simulink model "positionControlBalancing"  (Simulink 9.0)
settings: Solver=FixedStepDiscrete  StartTime=0.0  StopTime="Config.SIMULATION_TIME "  FixedStep=Config.tStep  RelTol=1e-3  EnableMultiTasking=on
PostLoadFcn:
  | %% Try to open the static GUI
  | try
  | 
  |     staticGUI = simulinkStaticGUI;
  | 
  | end
InitFcn:
  | %% initialize the simulation
  | cd(fileparts(which(bdroot)));
  | initPositionControlBalancing;
  | 
  | %% Try to edit the GUI (the user may have already closed it)
  | try
  | 
  |     %% Update Start Button
  |     set(sl_synch_handles.startButton,'Backgroundcolor',[0.0,1.0,0.0]);
  |     set(sl_synch_handles.startButton,'Enable','on');
  | 
  | end
StartFcn:
  | %% Try to edit the GUI (the user may have already closed it)
  | try
  | 
  |     %% Update Start Button
  |     set(sl_synch_handles.startButton,'Backgroundcolor',[0.8,0.8,0.8]);
  |     set(sl_synch_handles.startButton,'Enable','off');
  | 
  |     %% Update Compile Button
  |     set(sl_synch_handles.compileButton,'Backgroundcolor',[0.8,0.8,0.8]);
  |     set(sl_synch_handles.compileButton,'Enable','off');
  | 
  |     %% Update Exit Button
  |     set(sl_synch_handles.exitButton,'Backgroundcolor',[0.8,0.8,0.8]);
  |     set(sl_synch_handles.exitButton,'Enable','off');
  | 
  | end
StopFcn:
  | %% stop the simulation
  | cd(fileparts(which(bdroot)));
  | stopPositionControlBalancing;
  | 
  | %% Try to edit the GUI (the user may have already closed it)
  | try
  | 
  |     %% Update Compile Button
  |     set(sl_synch_handles.compileButton,'Backgroundcolor',[1.0,0.6,0.0]);
  |     set(sl_synch_handles.compileButton,'Enable','on');
  | 
  |     %% Update Exit Button
  |     set(sl_synch_handles.exitButton,'Backgroundcolor',[0.0,1.0,1.0]);
  |     set(sl_synch_handles.exitButton,'Enable','on');
  | 
  | end
undefined symbols (not defined in the file or in its folder): Config, DiscIntNeverNeededParam, ROBOT_DOF, Sat
libraries: WBToolboxLibrary x28
CloseFcn:
  | %% Try to close the GUI (the user might have already closed it)
  | try
  | 
  |     close(simulinkStaticGUI)
  | 
  | end
settings Model: SuppressorTable=22 serialization::archive 11 0 6 0 0 0 1 0  Creator=daniele  LastModifiedBy=gnava
settings DataIOCC: LimitDataPoints=on
settings OptimizationCC: ExpressionDepthLimit=2147483647
settings DebuggingCC: SolverPrmCheckMsg=warning  FcnCallInpInsideContextMsg=warning  AllowSymbolicDim=off  StateNameClashWarn=warning
settings SFSimCC: SimParseCustomCode=off
settings RTWCC: GenCodeOnly=on  TargetLang=C++
settings GRTTargetCC: TargetLangStandard=C++03 (ISO)  GeneratePreprocessorConditionals=Disable all  MatFileLogging=off  MultiInstanceERTCode=on  CodeInterfacePackaging=C++ class  SupportNonFinite=off
settings CPPComponent: GenerateDestructor=on  GenerateExternalIOAccessMethods=None  ParameterMemberVisibility=private  InternalMemberVisibility=private  GenerateParameterAccessMethods=None  GenerateInternalMemberAccessMethods=None  UseOperatorNewForModelRefRegistration=off

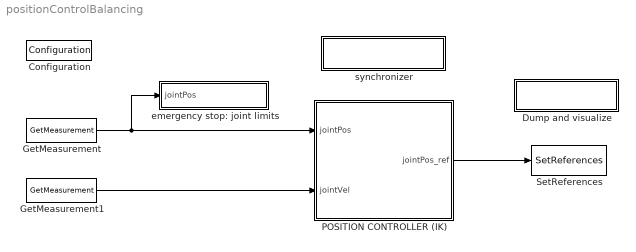
== system positionControlBalancing ==
  Configuration : WBToolboxLibrary/Utilities/Configuration  ConfigSource=Workspace  ConfigObject='WBTConfigRobot'  RobotName='icubSim'  UrdfFile='model.urdf'  ControlledJoints={'l_elbow','l_shoulder_pitch','torso_roll'}  ControlBoardsNames={'left_arm','right_arm','torso'}  LocalName='WBT'  GravityVector=[0,0,-9.81]
      settings: SourceProductName=WholeBodyToolbox
  Dump and visualize : Subsystem
      mask Display: disp('VISUALIZER')
  GetMeasurement : WBToolboxLibrary/States/GetMeasurement  measuredType=Joints Position
      settings: SourceProductName=WholeBodyToolbox
  GetMeasurement1 : WBToolboxLibrary/States/GetMeasurement  measuredType=Joints Velocity
      settings: SourceProductName=WholeBodyToolbox
  POSITION CONTROLLER (IK) : Subsystem
  SetReferences : WBToolboxLibrary/Actuators/SetReferences  controlType=Position Direct  refSpeed=10*(pi/180)  refAcceleration=1000000*(pi/180)
      settings: SourceProductName=WholeBodyToolbox
  emergency stop: joint limits : Subsystem
      mask Display: disp('EMERGENCY STOP')
  synchronizer : Subsystem
      mask Display: disp('SYNCHRONIZER')
  wires:
  POSITION CONTROLLER (IK)/1(jointPos_ref) -> SetReferences/1
  GetMeasurement/1 -> POSITION CONTROLLER (IK)/1(jointPos), emergency stop: joint limits/1(jointPos)
  GetMeasurement1/1 -> POSITION CONTROLLER (IK)/2(jointVel)

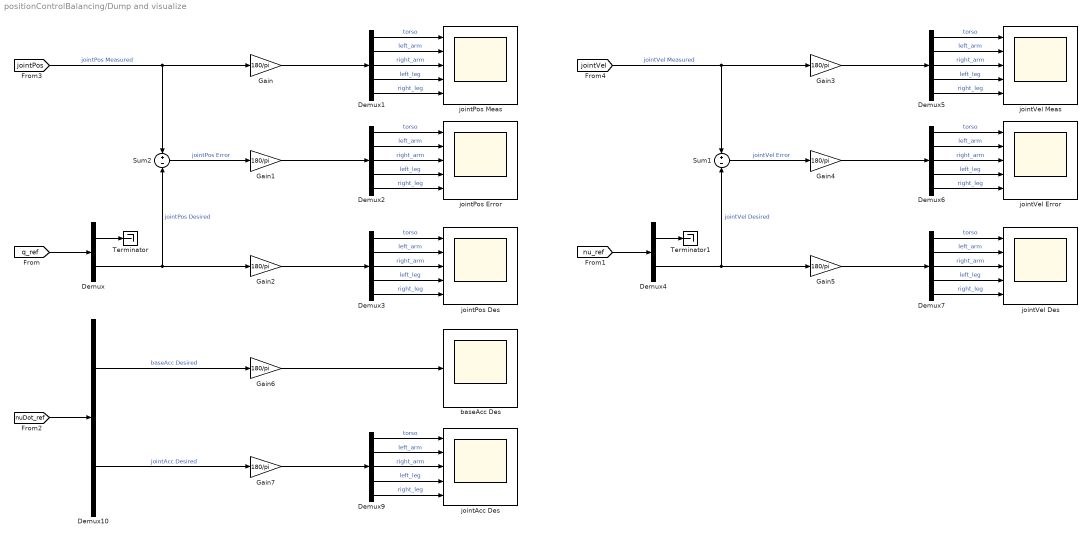
== system positionControlBalancing/Dump and visualize ==
  Demux : Demux  Outputs=[16;ROBOT_DOF]
  Demux{1..3,5..7,9} (7 alike) : Demux  Outputs=Config.numOfJointsForEachControlboard
  Demux10 : Demux  Outputs=[6;ROBOT_DOF]
  Demux4 : Demux  Outputs=[6;ROBOT_DOF]
  Gain{,1..7} (8 alike) : Gain  Gain=180/pi
  Sum1 : Sum  Inputs=+|-
  Sum2 : Sum  Inputs=+|-
  Terminator : Terminator
  Terminator1 : Terminator
  baseAcc Des : Scope
  jointAcc Des : Scope  NumInputPorts=5
  jointPos Des : Scope  NumInputPorts=5
  jointPos Error : Scope  NumInputPorts=5
  jointPos Meas : Scope  NumInputPorts=5
  jointVel Des : Scope  NumInputPorts=5
  jointVel Error : Scope  NumInputPorts=5
  jointVel Meas : Scope  NumInputPorts=5
  wires:
  Demux3/4 -> jointPos Des/4  "left_leg"
  Gain2/1 -> Demux3/1
  Demux2/5 -> jointPos Error/5  "right_leg"
  Demux2/4 -> jointPos Error/4  "left_leg"
  Demux3/1 -> jointPos Des/1  "torso"
  Demux3/5 -> jointPos Des/5  "right_leg"
  Demux1/3 -> jointPos Meas/3  "right_arm"
  Demux/2 -> Gain2/1, Sum2/2  "jointPos Desired"
  Gain1/1 -> Demux2/1
  Demux1/5 -> jointPos Meas/5  "right_leg"
  Demux1/1 -> jointPos Meas/1  "torso"
  Demux2/1 -> jointPos Error/1  "torso"
  Demux2/2 -> jointPos Error/2  "left_arm"
  Demux2/3 -> jointPos Error/3  "right_arm"
  Demux3/3 -> jointPos Des/3  "right_arm"
  Demux3/2 -> jointPos Des/2  "left_arm"
  Sum2/1 -> Gain1/1  "jointPos Error"
  Demux1/2 -> jointPos Meas/2  "left_arm"
  Gain/1 -> Demux1/1
  [jointPos] -> Sum2/1, Gain/1  "jointPos Measured"
  Demux1/4 -> jointPos Meas/4  "left_leg"
  [q_ref] -> Demux/1
  Demux/1 -> Terminator/1
  Demux4/1 -> Terminator1/1
  Demux6/2 -> jointVel Error/2  "left_arm"
  Demux6/3 -> jointVel Error/3  "right_arm"
  [jointVel] -> Sum1/1, Gain3/1  "jointVel Measured"
  Demux7/5 -> jointVel Des/5  "right_leg"
  Demux5/1 -> jointVel Meas/1  "torso"
  Demux7/4 -> jointVel Des/4  "left_leg"
  Demux6/4 -> jointVel Error/4  "left_leg"
  Sum1/1 -> Gain4/1  "jointVel Error"
  Demux7/3 -> jointVel Des/3  "right_arm"
  Demux4/2 -> Gain5/1, Sum1/2  "jointVel Desired"
  Demux6/5 -> jointVel Error/5  "right_leg"
  Demux5/2 -> jointVel Meas/2  "left_arm"
  Gain3/1 -> Demux5/1
  Demux5/3 -> jointVel Meas/3  "right_arm"
  [nu_ref] -> Demux4/1
  Demux7/1 -> jointVel Des/1  "torso"
  Demux6/1 -> jointVel Error/1  "torso"
  Gain5/1 -> Demux7/1
  Demux5/5 -> jointVel Meas/5  "right_leg"
  Gain4/1 -> Demux6/1
  Demux7/2 -> jointVel Des/2  "left_arm"
  Demux5/4 -> jointVel Meas/4  "left_leg"
  Demux10/1 -> Gain6/1  "baseAcc Desired"
  Gain7/1 -> Demux9/1
  Demux9/4 -> jointAcc Des/4  "left_leg"
  Demux9/3 -> jointAcc Des/3  "right_arm"
  Demux9/2 -> jointAcc Des/2  "left_arm"
  Demux9/5 -> jointAcc Des/5  "right_leg"
  Demux9/1 -> jointAcc Des/1  "torso"
  Demux10/2 -> Gain7/1  "jointAcc Desired"
  [nuDot_ref] -> Demux10/1
  Gain6/1 -> baseAcc Des/1

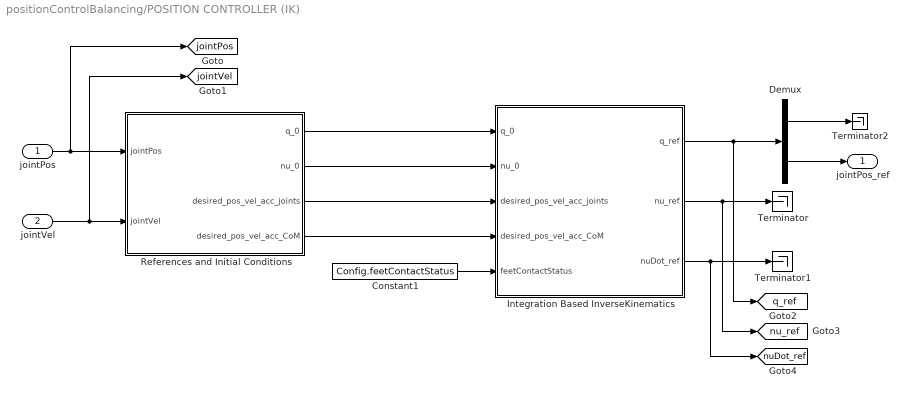
== system positionControlBalancing/POSITION CONTROLLER (IK) ==
  jointPos : Inport
  jointVel : Inport  Port=2
  Constant1 : Constant  Value=Config.feetContactStatus
  Demux : Demux  Outputs=[16;ROBOT_DOF]
  Integration Based InverseKinematics : Subsystem
  References and Initial Conditions : Subsystem
  Terminator : Terminator
  Terminator1 : Terminator
  Terminator2 : Terminator
  jointPos_ref : Outport
  tag scope: jointPos=global, jointVel=global, nuDot_ref=global, nu_ref=global, q_ref=global
  wires:
  jointPos/1 -> [jointPos], References and Initial Conditions/1(jointPos)
  jointVel/1 -> [jointVel], References and Initial Conditions/2(jointVel)
  References and Initial Conditions/1(q_0) -> Integration Based InverseKinematics/1(q_0)
  References and Initial Conditions/2(nu_0) -> Integration Based InverseKinematics/2(nu_0)
  References and Initial Conditions/3(desired_pos_vel_acc_joints) -> Integration Based InverseKinematics/3(desired_pos_vel_acc_joints)
  References and Initial Conditions/4(desired_pos_vel_acc_CoM) -> Integration Based InverseKinematics/4(desired_pos_vel_acc_CoM)
  Constant1/1 -> Integration Based InverseKinematics/5(feetContactStatus)
  Integration Based InverseKinematics/2(nu_ref) -> [nu_ref], Terminator/1
  Integration Based InverseKinematics/3(nuDot_ref) -> [nuDot_ref], Terminator1/1
  Integration Based InverseKinematics/1(q_ref) -> [q_ref], Demux/1
  Demux/1 -> Terminator2/1
  Demux/2 -> jointPos_ref/1

== system positionControlBalancing/emergency stop: joint limits ==
  jointPos : Inport
  ON_GAZEBO 1 : Constant  Value=Config.EMERGENCY_STOP_WITH_JOINTS_LIMITS
  ON_GAZEBO 2 : Constant  Value=Config.EMERGENCY_STOP_WITH_ENCODER_SPIKES
  STOP IF JOINTS HIT THE LIMITS : Subsystem
  STOP IF THERE ARE SPIKES IN THE ENCODERS : Subsystem
  wires:
  ON_GAZEBO 1/1 -> STOP IF JOINTS HIT THE LIMITS/Enable
  jointPos/1 -> STOP IF THERE ARE SPIKES IN THE ENCODERS/1(jointPos), STOP IF JOINTS HIT THE LIMITS/1(jointPos)
  ON_GAZEBO 2/1 -> STOP IF THERE ARE SPIKES IN THE ENCODERS/Enable

== system positionControlBalancing/synchronizer ==
  GAZEBO_SYNCHRONIZER : Subsystem
  Logical Operator : Logic  Operator=NOT  AllPortsSameDT=off  OutDataTypeStr=boolean
  "ON_GAZEBO " : Constant  Value=Config.ON_GAZEBO
  REAL_TIME_SYNC : Subsystem
  To Workspace : ToWorkspace  VariableName=yarp_time  SaveFormat=Structure With Time  SampleTime=-1
  Yarp Clock : WBToolboxLibrary/Utilities/Yarp Clock
      settings: SourceProductName=WholeBodyToolbox
  wires:
  Logical Operator/1 -> REAL_TIME_SYNC/Enable
  "ON_GAZEBO "/1 -> GAZEBO_SYNCHRONIZER/Enable, Logical Operator/1
  Yarp Clock/1 -> To Workspace/1

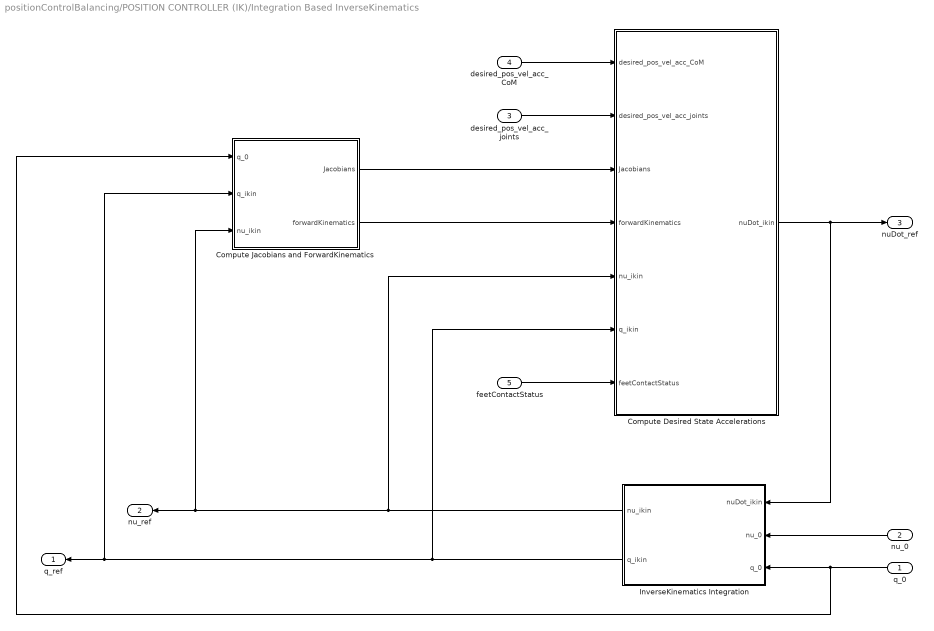
== system positionControlBalancing/POSITION CONTROLLER (IK)/Integration Based InverseKinematics ==
  q_0 : Inport
  nu_0 : Inport  Port=2
  desired_pos_vel_acc_joints : Inport  Port=3
  desired_pos_vel_acc_CoM : Inport  Port=4
  feetContactStatus : Inport  Port=5
  Compute Desired State Accelerations : Subsystem
  Compute Jacobians and ForwardKinematics : Subsystem
  InverseKinematics Integration : Subsystem
  q_ref : Outport
  nu_ref : Outport  Port=2
  nuDot_ref : Outport  Port=3
  wires:
  desired_pos_vel_acc_CoM/1 -> Compute Desired State Accelerations/1(desired_pos_vel_acc_CoM)
  desired_pos_vel_acc_joints/1 -> Compute Desired State Accelerations/2(desired_pos_vel_acc_joints)
  q_0/1 -> Compute Jacobians and ForwardKinematics/1(q_0), InverseKinematics Integration/3(q_0)
  InverseKinematics Integration/2(q_ikin) -> q_ref/1, Compute Jacobians and ForwardKinematics/2(q_ikin), Compute Desired State Accelerations/6(q_ikin)
  Compute Jacobians and ForwardKinematics/1(Jacobians) -> Compute Desired State Accelerations/3(Jacobians)
  Compute Jacobians and ForwardKinematics/2(forwardKinematics) -> Compute Desired State Accelerations/4(forwardKinematics)
  Compute Desired State Accelerations/1(nuDot_ikin) -> InverseKinematics Integration/1(nuDot_ikin), nuDot_ref/1
  feetContactStatus/1 -> Compute Desired State Accelerations/7(feetContactStatus)
  nu_0/1 -> InverseKinematics Integration/2(nu_0)
  InverseKinematics Integration/1(nu_ikin) -> nu_ref/1, Compute Jacobians and ForwardKinematics/3(nu_ikin), Compute Desired State Accelerations/5(nu_ikin)

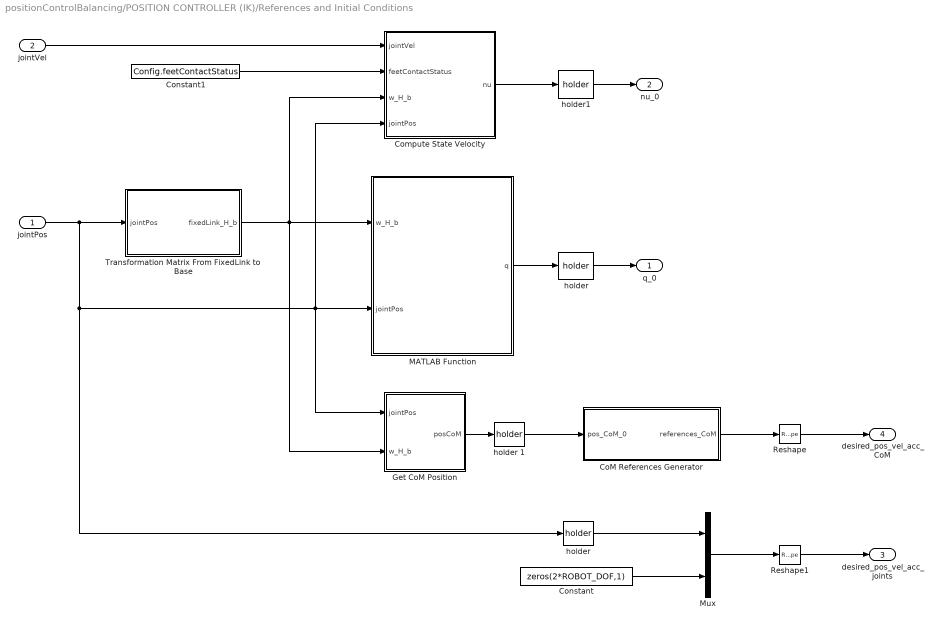
== system positionControlBalancing/POSITION CONTROLLER (IK)/References and Initial Conditions ==
  jointPos : Inport
  jointVel : Inport  Port=2
  CoM References Generator : Subsystem
  Compute State Velocity : Subsystem
  Constant : Constant  Value=zeros(2*ROBOT_DOF,1)
  Constant1 : Constant  Value=Config.feetContactStatus
  Get CoM Position : Subsystem
  MATLAB Function : MATLAB Function  TreatAsAtomicUnit=on
  Mux : Mux  Inputs=2
  Reshape : Reshape  OutputDimensionality=Customize  OutputDimensions=[3,3]
  Reshape1 : Reshape  OutputDimensionality=Customize  OutputDimensions=[ROBOT_DOF,3]
  Transformation Matrix From FixedLink to Base : Subsystem
  holder : WBToolboxLibrary/Utilities/holder 
      settings: SourceProductName=WholeBodyToolbox
  "holder " : WBToolboxLibrary/Utilities/holder 
      settings: SourceProductName=WholeBodyToolbox
  holder 1 : WBToolboxLibrary/Utilities/holder 
      settings: SourceProductName=WholeBodyToolbox
  holder1 : WBToolboxLibrary/Utilities/holder 
      settings: SourceProductName=WholeBodyToolbox
  q_0 : Outport
  nu_0 : Outport  Port=2
  desired_pos_vel_acc_joints : Outport  Port=3
  desired_pos_vel_acc_CoM : Outport  Port=4
  wires:
  CoM References Generator/1(references_CoM) -> Reshape/1
  Compute State Velocity/1(nu) -> holder1/1
  Get CoM Position/1(posCoM) -> holder 1/1
  Constant1/1 -> Compute State Velocity/2("feetContactStatus ")
  Reshape/1 -> desired_pos_vel_acc_CoM/1
  holder 1/1 -> CoM References Generator/1(pos_CoM_0)
  Transformation Matrix From FixedLink to Base/1(fixedLink_H_b) -> Get CoM Position/2(w_H_b), Compute State Velocity/3(w_H_b), MATLAB Function/1(w_H_b)
  MATLAB Function/1(q) -> holder/1
  jointPos/1 -> Transformation Matrix From FixedLink to Base/1(jointPos), "holder "/1, Get CoM Position/1(jointPos), Compute State Velocity/4(jointPos), MATLAB Function/2(jointPos)
  holder/1 -> q_0/1
  jointVel/1 -> Compute State Velocity/1(jointVel)
  holder1/1 -> nu_0/1
  Constant/1 -> Mux/2
  "holder "/1 -> Mux/1
  Mux/1 -> Reshape1/1
  Reshape1/1 -> desired_pos_vel_acc_joints/1

== system positionControlBalancing/emergency stop: joint limits/STOP IF JOINTS HIT THE LIMITS ==
  jointPos : Inport
  Enable : EnablePort
  Assertion : Assertion
  GetLimits : WBToolboxLibrary/States/GetLimits  limitsSource=ControlBoard  limitsType=Position
      settings: SourceProductName=WholeBodyToolbox
  MATLAB Function : MATLAB Function  TreatAsAtomicUnit=on
  index1 : Constant  Value=0.01  VectorParams1D=off
  wires:
  jointPos/1 -> MATLAB Function/3(u)
  MATLAB Function/1(inRange) -> Assertion/1
  GetLimits/1 -> MATLAB Function/1(umin)
  GetLimits/2 -> MATLAB Function/2(umax)
  index1/1 -> MATLAB Function/4(tol)

== system positionControlBalancing/emergency stop: joint limits/STOP IF THERE ARE SPIKES IN THE ENCODERS ==
  jointPos : Inport
  Enable : EnablePort
  Assertion : Assertion
  MATLAB Function : MATLAB Function  TreatAsAtomicUnit=on
  index1 : Constant  Value=Sat.maxJointsPositionDelta  VectorParams1D=off
  wires:
  jointPos/1 -> MATLAB Function/1(u)
  MATLAB Function/1(noSpikes) -> Assertion/1
  index1/1 -> MATLAB Function/2(delta_u_max)

== system positionControlBalancing/synchronizer/GAZEBO_SYNCHRONIZER ==
  Enable : EnablePort
  Simulator Synchronizer : WBToolboxLibrary/Utilities/Simulator Synchronizer  period=Config.tStep  serverPortName='/clock/rpc'  clientPortName='/WBT_synchronizer/rpc:o'
      settings: SourceProductName=WholeBodyToolbox

== system positionControlBalancing/synchronizer/REAL_TIME_SYNC ==
  Enable : EnablePort
  Real Time Synchronizer : WBToolboxLibrary/Utilities/Real Time Synchronizer  period=Config.tStep
      settings: SourceProductName=WholeBodyToolbox

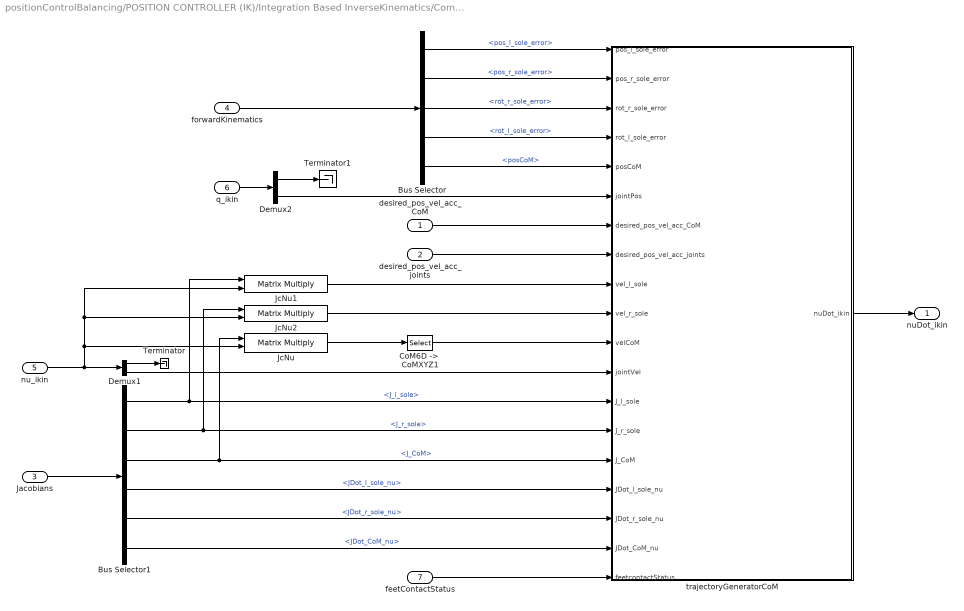
== system positionControlBalancing/POSITION CONTROLLER (IK)/Integration Based InverseKinematics/Compute Desired State Accelerations ==
  desired_pos_vel_acc_CoM : Inport
  desired_pos_vel_acc_joints : Inport  Port=2
  Jacobians : Inport  Port=3
  forwardKinematics : Inport  Port=4
  nu_ikin : Inport  Port=5
  q_ikin : Inport  Port=6
  feetContactStatus : Inport  Port=7
  Bus Selector : BusSelector  OutputSignals=pos_l_sole_error,pos_r_sole_error,rot_r_sole_error,rot_l_sole_error,posCoM
  Bus Selector1 : BusSelector  OutputSignals=J_l_sole,J_r_sole,J_CoM,JDot_l_sole_nu,JDot_r_sole_nu,JDot_CoM_nu
  "CoM6D ->  CoMXYZ1" : Selector  InputPortWidth=6  IndexOptions=Index vector (dialog)  Indices=[1 2 3]  OutputSizes=1
  Demux1 : Demux  Outputs=[6,ROBOT_DOF]
  Demux2 : Demux  Outputs=[16,ROBOT_DOF]
  JcNu : Product  Multiplication=Matrix(*)
  JcNu1 : Product  Multiplication=Matrix(*)
  JcNu2 : Product  Multiplication=Matrix(*)
  Terminator : Terminator
  Terminator1 : Terminator
  trajectoryGeneratorCoM : MATLAB Function  TreatAsAtomicUnit=on
  nuDot_ikin : Outport
  wires:
  Demux1/1 -> Terminator/1
  JcNu/1 -> "CoM6D ->  CoMXYZ1"/1
  q_ikin/1 -> Demux2/1
  Demux2/1 -> Terminator1/1
  trajectoryGeneratorCoM/1(nuDot_ikin) -> nuDot_ikin/1
  desired_pos_vel_acc_CoM/1 -> trajectoryGeneratorCoM/7(desired_pos_vel_acc_CoM)
  desired_pos_vel_acc_joints/1 -> trajectoryGeneratorCoM/8(desired_pos_vel_acc_joints)
  feetContactStatus/1 -> trajectoryGeneratorCoM/19(feetcontactStatus)
  nu_ikin/1 -> JcNu1/2, JcNu2/2, JcNu/2, Demux1/1
  forwardKinematics/1 -> Bus Selector/1
  Bus Selector/1 -> trajectoryGeneratorCoM/1(pos_l_sole_error)  "<pos_l_sole_error>"
  Bus Selector/2 -> trajectoryGeneratorCoM/2(pos_r_sole_error)  "<pos_r_sole_error>"
  Bus Selector/3 -> trajectoryGeneratorCoM/3(rot_r_sole_error)  "<rot_r_sole_error>"
  Bus Selector/4 -> trajectoryGeneratorCoM/4(rot_l_sole_error)  "<rot_l_sole_error>"
  Bus Selector/5 -> trajectoryGeneratorCoM/5(posCoM)  "<posCoM>"
  Demux2/2 -> trajectoryGeneratorCoM/6(jointPos)
  Jacobians/1 -> Bus Selector1/1
  Bus Selector1/1 -> JcNu1/1, trajectoryGeneratorCoM/13(J_l_sole)  "<J_l_sole>"
  Bus Selector1/2 -> JcNu2/1, trajectoryGeneratorCoM/14(J_r_sole)  "<J_r_sole>"
  Bus Selector1/3 -> JcNu/1, trajectoryGeneratorCoM/15(J_CoM)  "<J_CoM>"
  Bus Selector1/4 -> trajectoryGeneratorCoM/16(JDot_l_sole_nu)  "<JDot_l_sole_nu>"
  Bus Selector1/5 -> trajectoryGeneratorCoM/17(JDot_r_sole_nu)  "<JDot_r_sole_nu>"
  Bus Selector1/6 -> trajectoryGeneratorCoM/18(JDot_CoM_nu)  "<JDot_CoM_nu>"
  JcNu1/1 -> trajectoryGeneratorCoM/9(vel_l_sole)
  JcNu2/1 -> trajectoryGeneratorCoM/10(vel_r_sole)
  "CoM6D ->  CoMXYZ1"/1 -> trajectoryGeneratorCoM/11(velCoM)
  Demux1/2 -> trajectoryGeneratorCoM/12(jointVel)

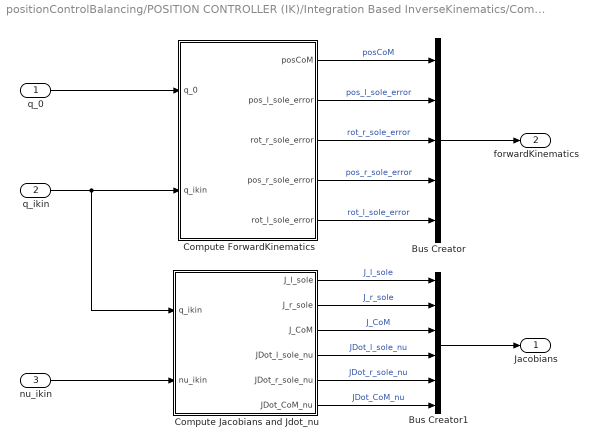
== system positionControlBalancing/POSITION CONTROLLER (IK)/Integration Based InverseKinematics/Compute Jacobians and ForwardKinematics ==
  q_0 : Inport
  q_ikin : Inport  Port=2
  nu_ikin : Inport  Port=3
  Bus Creator : BusCreator  Inputs=5
  Bus Creator1 : BusCreator  Inputs=6
  Compute ForwardKinematics : Subsystem
  Compute Jacobians and Jdot_nu : Subsystem
  Jacobians : Outport
  forwardKinematics : Outport  Port=2
  wires:
  q_0/1 -> Compute ForwardKinematics/1(q_0)
  q_ikin/1 -> Compute Jacobians and Jdot_nu/1(q_ikin), Compute ForwardKinematics/2(q_ikin)
  Compute ForwardKinematics/1(posCoM) -> Bus Creator/1  "posCoM"
  Compute ForwardKinematics/2(pos_l_sole_error) -> Bus Creator/2  "pos_l_sole_error"
  Compute ForwardKinematics/3(rot_r_sole_error) -> Bus Creator/3  "rot_r_sole_error"
  Compute ForwardKinematics/4(pos_r_sole_error) -> Bus Creator/4  "pos_r_sole_error"
  Compute ForwardKinematics/5(rot_l_sole_error) -> Bus Creator/5  "rot_l_sole_error"
  Bus Creator/1 -> forwardKinematics/1
  nu_ikin/1 -> Compute Jacobians and Jdot_nu/2(nu_ikin)
  Compute Jacobians and Jdot_nu/1(J_l_sole) -> Bus Creator1/1  "J_l_sole"
  Compute Jacobians and Jdot_nu/2(J_r_sole) -> Bus Creator1/2  "J_r_sole"
  Compute Jacobians and Jdot_nu/3(J_CoM) -> Bus Creator1/3  "J_CoM"
  Compute Jacobians and Jdot_nu/4(JDot_l_sole_nu) -> Bus Creator1/4  "JDot_l_sole_nu"
  Compute Jacobians and Jdot_nu/5(JDot_r_sole_nu) -> Bus Creator1/5  "JDot_r_sole_nu"
  Compute Jacobians and Jdot_nu/6(JDot_CoM_nu) -> Bus Creator1/6  "JDot_CoM_nu"
  Bus Creator1/1 -> Jacobians/1

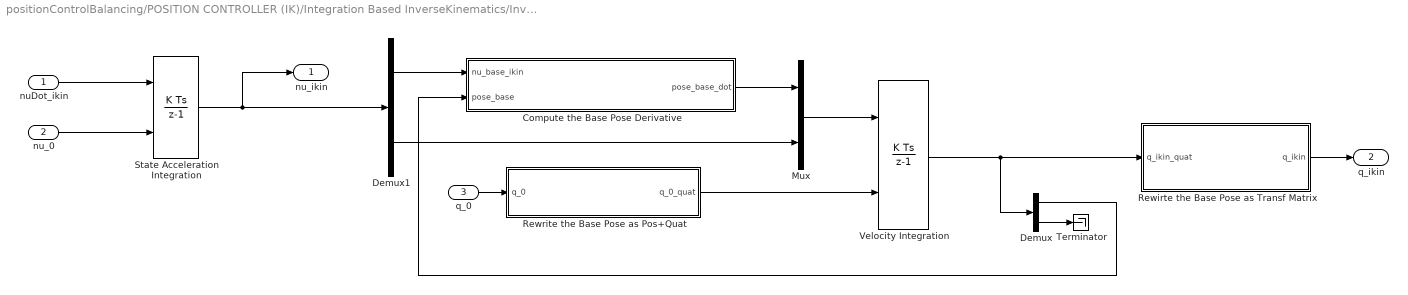
== system positionControlBalancing/POSITION CONTROLLER (IK)/Integration Based InverseKinematics/InverseKinematics Integration ==
  nuDot_ikin : Inport
  nu_0 : Inport  Port=2
  q_0 : Inport  Port=3
  Compute the Base Pose Derivative : MATLAB Function  TreatAsAtomicUnit=on
  Demux : Demux  Outputs=[7;ROBOT_DOF]
  Demux1 : Demux  Outputs=[6;ROBOT_DOF]
  Mux : Mux  Inputs=2
  Rewirte the Base Pose as Transf Matrix : MATLAB Function  TreatAsAtomicUnit=on
  Rewrite the Base Pose as Pos+Quat : MATLAB Function  TreatAsAtomicUnit=on
  State Acceleration Integration : DiscreteIntegrator  InitialConditionSource=external  SampleTime=Config.tStep  ICPrevOutput=DiscIntNeverNeededParam  ICPrevScaledInput=DiscIntNeverNeededParam
  Terminator : Terminator
  Velocity Integration : DiscreteIntegrator  InitialConditionSource=external  SampleTime=Config.tStep  ICPrevOutput=DiscIntNeverNeededParam  ICPrevScaledInput=DiscIntNeverNeededParam
  nu_ikin : Outport
  q_ikin : Outport  Port=2
  wires:
  nu_0/1 -> State Acceleration Integration/2
  q_0/1 -> Rewrite the Base Pose as Pos+Quat/1(q_0)
  nuDot_ikin/1 -> State Acceleration Integration/1
  Demux/2 -> Terminator/1
  Velocity Integration/1 -> Demux/1, Rewirte the Base Pose as Transf Matrix/1(q_ikin_quat)
  State Acceleration Integration/1 -> Demux1/1, nu_ikin/1
  Demux1/1 -> Compute the Base Pose Derivative/1(nu_base_ikin)
  Compute the Base Pose Derivative/1(pose_base_dot) -> Mux/1
  Demux1/2 -> Mux/2
  Mux/1 -> Velocity Integration/1
  Rewirte the Base Pose as Transf Matrix/1(q_ikin) -> q_ikin/1
  Rewrite the Base Pose as Pos+Quat/1(q_0_quat) -> Velocity Integration/2
  Demux/1 -> Compute the Base Pose Derivative/2(pose_base)

== system positionControlBalancing/POSITION CONTROLLER (IK)/References and Initial Conditions/CoM References Generator ==
  pos_CoM_0 : Inport
  Clock1 : Clock
  Constant : Constant  Value=Config.COM_SINE_MOVEMENTS
  Constant2 : Constant  Value=zeros(6,1)
  Mux : Mux  Inputs=2
  Reference Generator CoM : MATLAB Function  TreatAsAtomicUnit=on
  Switch1 : Switch  Criteria=u2 > Threshold
  references_CoM : Outport
  wires:
  Clock1/1 -> Reference Generator CoM/2(t)
  Constant2/1 -> Mux/2
  pos_CoM_0/1 -> Reference Generator CoM/1(posCoM_0), Mux/1
  Constant/1 -> Switch1/2
  Mux/1 -> Switch1/3
  Reference Generator CoM/1(references_CoM) -> Switch1/1
  Switch1/1 -> references_CoM/1

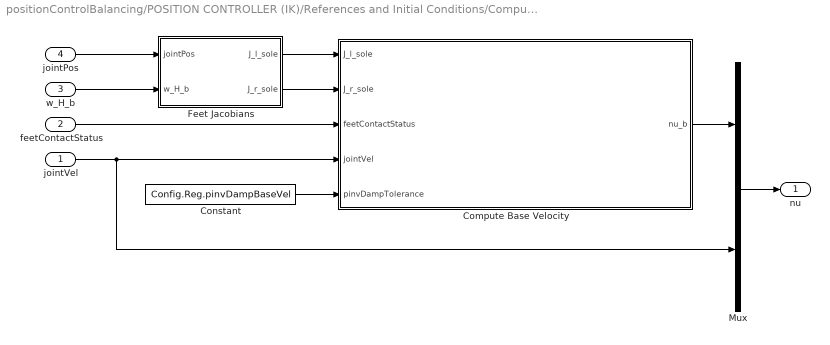
== system positionControlBalancing/POSITION CONTROLLER (IK)/References and Initial Conditions/Compute State Velocity ==
  jointVel : Inport
  "feetContactStatus " : Inport  Port=2
  w_H_b : Inport  Port=3
  jointPos : Inport  Port=4
  Compute Base Velocity : MATLAB Function  TreatAsAtomicUnit=on
  Constant : Constant  Value=Config.Reg.pinvDampBaseVel
  Feet Jacobians : Subsystem
  Mux : Mux  Inputs=2
  nu : Outport
  wires:
  Mux/1 -> nu/1
  "feetContactStatus "/1 -> Compute Base Velocity/3(feetContactStatus)
  Compute Base Velocity/1(nu_b) -> Mux/1
  jointPos/1 -> Feet Jacobians/1(jointPos)
  w_H_b/1 -> Feet Jacobians/2(w_H_b)
  Feet Jacobians/1(J_l_sole) -> Compute Base Velocity/1(J_l_sole)
  Feet Jacobians/2(J_r_sole) -> Compute Base Velocity/2(J_r_sole)
  jointVel/1 -> Compute Base Velocity/4(jointVel), Mux/2
  Constant/1 -> Compute Base Velocity/5(pinvDampTolerance)

== system positionControlBalancing/POSITION CONTROLLER (IK)/References and Initial Conditions/Get CoM Position ==
  jointPos : Inport
  w_H_b : Inport  Port=2
  CoM Position : WBToolboxLibrary/Model/Kinematics/ForwardKinematics  frameName=Frames.COM
      settings: SourceProductName=WholeBodyToolbox
  "CoM6D ->  CoMXYZ2" : Selector  NumberOfDimensions=2  InputPortWidth=7  IndexOptions=Index vector (dialog),Index vector (dialog)  Indices=[1 2 3],[4]  OutputSizes=1,1
  posCoM : Outport
  wires:
  jointPos/1 -> CoM Position/2
  "CoM6D ->  CoMXYZ2"/1 -> posCoM/1
  CoM Position/1 -> "CoM6D ->  CoMXYZ2"/1
  w_H_b/1 -> CoM Position/1

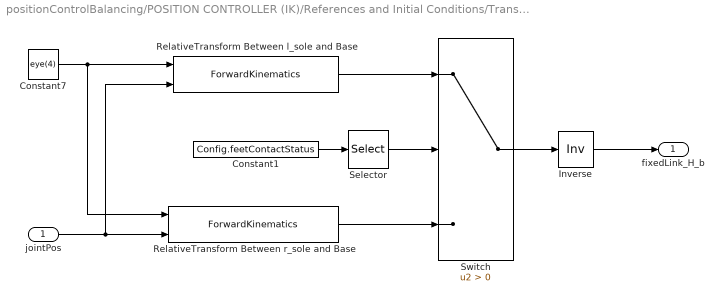
== system positionControlBalancing/POSITION CONTROLLER (IK)/References and Initial Conditions/Transformation Matrix From FixedLink to Base ==
  jointPos : Inport
  Constant1 : Constant  Value=Config.feetContactStatus
  Constant7 : Constant  Value=eye(4)
  "Inverse  " : Product  Inputs=/  Multiplication=Matrix(*)
  RelativeTransform Between l_sole and Base : WBToolboxLibrary/Model/Kinematics/ForwardKinematics  frameName=Frames.LEFT_FOOT
      settings: SourceProductName=WholeBodyToolbox
  RelativeTransform Between r_sole and Base : WBToolboxLibrary/Model/Kinematics/ForwardKinematics  frameName=Frames.RIGHT_FOOT
      settings: SourceProductName=WholeBodyToolbox
  Selector : Selector  InputPortWidth=2  IndexOptions=Index vector (dialog)  Indices=1  OutputSizes=1
  Switch : Switch  Criteria=u2 > Threshold
  fixedLink_H_b : Outport
  wires:
  jointPos/1 -> RelativeTransform Between l_sole and Base/2, RelativeTransform Between r_sole and Base/2
  Constant7/1 -> RelativeTransform Between r_sole and Base/1, RelativeTransform Between l_sole and Base/1
  RelativeTransform Between l_sole and Base/1 -> Switch/1
  RelativeTransform Between r_sole and Base/1 -> Switch/3
  Constant1/1 -> Selector/1
  Switch/1 -> "Inverse  "/1
  "Inverse  "/1 -> fixedLink_H_b/1
  Selector/1 -> Switch/2

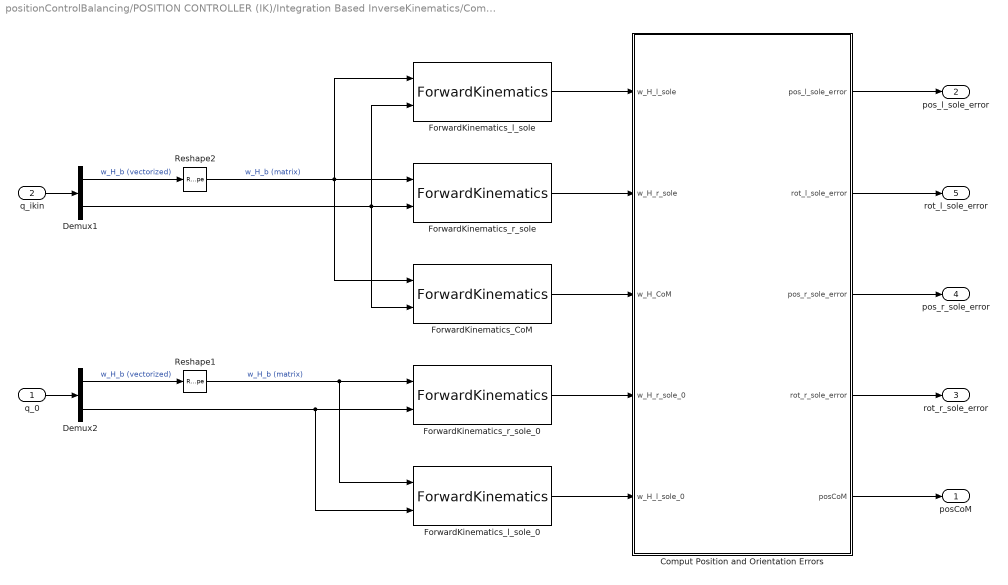
== system positionControlBalancing/POSITION CONTROLLER (IK)/Integration Based InverseKinematics/Compute Jacobians and ForwardKinematics/Compute ForwardKinematics ==
  q_0 : Inport
  q_ikin : Inport  Port=2
  Comput Position and Orientation Errors : MATLAB Function  TreatAsAtomicUnit=on
  Demux1 : Demux  Outputs=[16;ROBOT_DOF]
  Demux2 : Demux  Outputs=[16;ROBOT_DOF]
  ForwardKinematics_CoM : WBToolboxLibrary/Model/Kinematics/ForwardKinematics  frameName=Frames.COM
      settings: SourceProductName=WholeBodyToolbox
  ForwardKinematics_l_sole : WBToolboxLibrary/Model/Kinematics/ForwardKinematics  frameName=Frames.LEFT_FOOT
      settings: SourceProductName=WholeBodyToolbox
  ForwardKinematics_l_sole_0 : WBToolboxLibrary/Model/Kinematics/ForwardKinematics  frameName=Frames.LEFT_FOOT
      settings: SourceProductName=WholeBodyToolbox
  ForwardKinematics_r_sole : WBToolboxLibrary/Model/Kinematics/ForwardKinematics  frameName=Frames.RIGHT_FOOT
      settings: SourceProductName=WholeBodyToolbox
  ForwardKinematics_r_sole_0 : WBToolboxLibrary/Model/Kinematics/ForwardKinematics  frameName=Frames.RIGHT_FOOT
      settings: SourceProductName=WholeBodyToolbox
  Reshape1 : Reshape  OutputDimensionality=Customize  OutputDimensions=[4,4]
  Reshape2 : Reshape  OutputDimensionality=Customize  OutputDimensions=[4,4]
  posCoM : Outport
  pos_l_sole_error : Outport  Port=2
  rot_r_sole_error : Outport  Port=3
  pos_r_sole_error : Outport  Port=4
  rot_l_sole_error : Outport  Port=5
  wires:
  q_0/1 -> Demux2/1
  Demux2/1 -> Reshape1/1  "w_H_b (vectorized)"
  q_ikin/1 -> Demux1/1
  Demux1/1 -> Reshape2/1  "w_H_b (vectorized)"
  Reshape2/1 -> ForwardKinematics_l_sole/1, ForwardKinematics_CoM/1, ForwardKinematics_r_sole/1  "w_H_b (matrix)"
  Reshape1/1 -> ForwardKinematics_r_sole_0/1, ForwardKinematics_l_sole_0/1  "w_H_b (matrix)"
  Demux2/2 -> ForwardKinematics_r_sole_0/2, ForwardKinematics_l_sole_0/2
  Demux1/2 -> ForwardKinematics_l_sole/2, ForwardKinematics_CoM/2, ForwardKinematics_r_sole/2
  ForwardKinematics_l_sole/1 -> Comput Position and Orientation Errors/1(w_H_l_sole)
  ForwardKinematics_r_sole/1 -> Comput Position and Orientation Errors/2(w_H_r_sole)
  ForwardKinematics_CoM/1 -> Comput Position and Orientation Errors/3(w_H_CoM)
  ForwardKinematics_r_sole_0/1 -> Comput Position and Orientation Errors/4(w_H_r_sole_0)
  ForwardKinematics_l_sole_0/1 -> Comput Position and Orientation Errors/5(w_H_l_sole_0)
  Comput Position and Orientation Errors/5(posCoM) -> posCoM/1
  Comput Position and Orientation Errors/1(pos_l_sole_error) -> pos_l_sole_error/1
  Comput Position and Orientation Errors/2(rot_l_sole_error) -> rot_l_sole_error/1
  Comput Position and Orientation Errors/3(pos_r_sole_error) -> pos_r_sole_error/1
  Comput Position and Orientation Errors/4(rot_r_sole_error) -> rot_r_sole_error/1

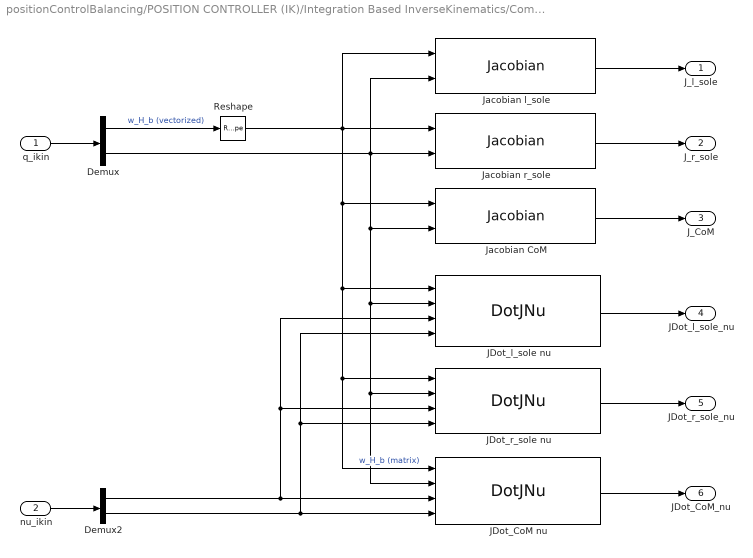
== system positionControlBalancing/POSITION CONTROLLER (IK)/Integration Based InverseKinematics/Compute Jacobians and ForwardKinematics/Compute Jacobians and Jdot_nu ==
  q_ikin : Inport
  nu_ikin : Inport  Port=2
  Demux : Demux  Outputs=[16;ROBOT_DOF]
  Demux2 : Demux  Outputs=[6;ROBOT_DOF]
  JDot_CoM nu : WBToolboxLibrary/Model/Jacobians/DotJNu  frameName=Frames.COM
      settings: SourceProductName=WholeBodyToolbox
  JDot_l_sole nu : WBToolboxLibrary/Model/Jacobians/DotJNu  frameName=Frames.LEFT_FOOT
      settings: SourceProductName=WholeBodyToolbox
  JDot_r_sole nu : WBToolboxLibrary/Model/Jacobians/DotJNu  frameName=Frames.RIGHT_FOOT
      settings: SourceProductName=WholeBodyToolbox
  Jacobian CoM : WBToolboxLibrary/Model/Jacobians/Jacobian  frameName=Frames.COM
      settings: SourceProductName=WholeBodyToolbox
  Jacobian l_sole : WBToolboxLibrary/Model/Jacobians/Jacobian  frameName=Frames.LEFT_FOOT
      settings: SourceProductName=WholeBodyToolbox
  Jacobian r_sole : WBToolboxLibrary/Model/Jacobians/Jacobian  frameName=Frames.RIGHT_FOOT
      settings: SourceProductName=WholeBodyToolbox
  Reshape : Reshape  OutputDimensionality=Customize  OutputDimensions=[4,4]
  J_l_sole : Outport
  J_r_sole : Outport  Port=2
  J_CoM : Outport  Port=3
  JDot_l_sole_nu : Outport  Port=4
  JDot_r_sole_nu : Outport  Port=5
  JDot_CoM_nu : Outport  Port=6
  wires:
  q_ikin/1 -> Demux/1
  Demux/1 -> Reshape/1  "w_H_b (vectorized)"
  Reshape/1 -> Jacobian r_sole/1, Jacobian l_sole/1, JDot_l_sole nu/1, JDot_r_sole nu/1, JDot_CoM nu/1, Jacobian CoM/1  "w_H_b (matrix)"
  Demux/2 -> Jacobian r_sole/2, JDot_CoM nu/2, JDot_r_sole nu/2, JDot_l_sole nu/2, Jacobian CoM/2, Jacobian l_sole/2
  Jacobian l_sole/1 -> J_l_sole/1
  Jacobian r_sole/1 -> J_r_sole/1
  Jacobian CoM/1 -> J_CoM/1
  Demux2/1 -> JDot_CoM nu/3, JDot_r_sole nu/3, JDot_l_sole nu/3
  Demux2/2 -> JDot_CoM nu/4, JDot_r_sole nu/4, JDot_l_sole nu/4
  JDot_l_sole nu/1 -> JDot_l_sole_nu/1
  JDot_r_sole nu/1 -> JDot_r_sole_nu/1
  nu_ikin/1 -> Demux2/1
  JDot_CoM nu/1 -> JDot_CoM_nu/1

== system positionControlBalancing/POSITION CONTROLLER (IK)/References and Initial Conditions/Compute State Velocity/Feet Jacobians ==
  jointPos : Inport
  w_H_b : Inport  Port=2
  Jacobian l_sole : WBToolboxLibrary/Model/Jacobians/Jacobian  frameName=Frames.LEFT_FOOT
      settings: SourceProductName=WholeBodyToolbox
  Jacobian r_sole : WBToolboxLibrary/Model/Jacobians/Jacobian  frameName=Frames.RIGHT_FOOT
      settings: SourceProductName=WholeBodyToolbox
  J_l_sole : Outport
  J_r_sole : Outport  Port=2
  wires:
  Jacobian l_sole/1 -> J_l_sole/1
  Jacobian r_sole/1 -> J_r_sole/1
  w_H_b/1 -> Jacobian r_sole/1, Jacobian l_sole/1
  jointPos/1 -> Jacobian l_sole/2, Jacobian r_sole/2

== matlab function POSITION CONTROLLER (IK)/Integration Based InverseKinematics/Compute Jacobians and ForwardKinematics/Compute ForwardKinematics/Comput Position and Orientation Errors ==
  data: w_H_l_sole input double; w_H_r_sole input double; w_H_CoM input double; w_H_r_sole_0 input double; pos_l_sole_error output double; w_H_l_sole_0 input double; rot_l_sole_error output double; pos_r_sole_error output double; rot_r_sole_error output double; posCoM output double
function [pos_l_sole_error, rot_l_sole_error, pos_r_sole_error, rot_r_sole_error, posCoM] = ...
             computePositionAndOrientationErrorsFCN(w_H_l_sole, w_H_r_sole, w_H_CoM, w_H_r_sole_0, w_H_l_sole_0)
         
    [pos_l_sole_error, rot_l_sole_error, pos_r_sole_error, rot_r_sole_error, posCoM] = ...
        computePositionAndOrientationErrors(w_H_l_sole, w_H_r_sole, w_H_CoM, w_H_r_sole_0, w_H_l_sole_0);
end

== matlab function POSITION CONTROLLER (IK)/References and Initial Conditions/Compute State Velocity/Compute Base Velocity ==
  data: J_l_sole input double; J_r_sole input double; feetContactStatus input double; nu_b output double; jointVel input double; pinvDampTolerance input double
function nu_b = computeBaseVelocityWithFeetContactFCN(J_l_sole, J_r_sole, feetContactStatus, jointVel, pinvDampTolerance)

    nu_b = wbc.computeBaseVelocityWithFeetContact(J_l_sole, J_r_sole, feetContactStatus, jointVel, pinvDampTolerance);
end

== matlab function POSITION CONTROLLER (IK)/References and Initial Conditions/CoM References Generator/Reference Generator CoM ==
  data: posCoM_0 input double; t input double; references_CoM output double; Config parameter double
function references_CoM = referenceGeneratorCoMFCN(posCoM_0, t, Config)

    references_CoM = referenceGeneratorCoM(posCoM_0, t, Config);
end

== matlab function emergency stop: joint limits/STOP IF THERE ARE SPIKES IN THE ENCODERS/MATLAB Function ==
  data: u input double; delta_u_max input double; noSpikes output double
function noSpikes = checkSpikes(u, delta_u_max)

     noSpikes = wbc.checkSpikes(u, delta_u_max);
end

== matlab function emergency stop: joint limits/STOP IF JOINTS HIT THE LIMITS/MATLAB Function ==
  data: umin input double; umax input double; u input double; inRange output double; tol input double
function inRange = checkRangeFCN(umin, umax, u, tol)

     inRange = wbc.checkRange(umin, umax, u, tol);
end

== matlab function POSITION CONTROLLER (IK)/Integration Based InverseKinematics/InverseKinematics Integration/Compute the Base Pose Derivative ==
  data: pose_base_dot output double; nu_base_ikin input double; pose_base input double
function pose_base_dot = computeBasePoseDerivativeFCN(nu_base_ikin, pose_base)

    pose_base_dot = computeBasePoseDerivative(nu_base_ikin, pose_base);
end

== matlab function POSITION CONTROLLER (IK)/References and Initial Conditions/MATLAB Function ==
  data: w_H_b input double; q output double; jointPos input double
function q = getSystemConfiguration(w_H_b,jointPos)

    q = [w_H_b(:);jointPos];
end

== matlab function POSITION CONTROLLER (IK)/Integration Based InverseKinematics/Compute Desired State Accelerations/trajectoryGeneratorCoM ==
  data: pos_l_sole_error input double; pos_r_sole_error input double; rot_r_sole_error input double; rot_l_sole_error input double; posCoM input double; jointPos input double; desired_pos_vel_acc_CoM input double; desired_pos_vel_acc_joints input double; vel_l_sole input double; vel_r_sole input double; velCoM input double; jointVel input double; J_l_sole input double; J_r_sole input double; J_CoM input double; JDot_l_sole_nu input double; JDot_r_sole_nu input double; JDot_CoM_nu input double; feetcontactStatus input double; nuDot_ikin output double; Config parameter double
function nuDot_ikin = computeStateAccelerationsFCN(pos_l_sole_error, pos_r_sole_error, rot_r_sole_error, rot_l_sole_error, ...
                                                   posCoM, jointPos, desired_pos_vel_acc_CoM, desired_pos_vel_acc_joints, vel_l_sole, vel_r_sole, ...
                                                   velCoM, jointVel, J_l_sole, J_r_sole, J_CoM, JDot_l_sole_nu, JDot_r_sole_nu, JDot_CoM_nu, feetcontactStatus, Config)
                                               
    nuDot_ikin = computeStateAccelerations(pos_l_sole_error, pos_r_sole_error, rot_r_sole_error, rot_l_sole_error, ...
                                           posCoM, jointPos, desired_pos_vel_acc_CoM, desired_pos_vel_acc_joints, vel_l_sole, vel_r_sole, ...
                                           velCoM, jointVel, J_l_sole, J_r_sole, J_CoM, JDot_l_sole_nu, JDot_r_sole_nu, JDot_CoM_nu, feetcontactStatus, Config);
end

== matlab function POSITION CONTROLLER (IK)/Integration Based InverseKinematics/InverseKinematics Integration/Rewrite the Base Pose as Pos+Quat ==
  data: q_0 input double; q_0_quat output double
function q_0_quat = fromTransfMatrixToQuaternions(q_0)

    % Reshape the base pose as a matrix
    w_H_base = [q_0(1:4) q_0(5:8) q_0(9:12) q_0(13:16)];

    % Get the base pos + quaternion
    qt_base  = wbc.fromTransfMatrixToPosQuat(w_H_base);

    % Final state converted as a 7+n element vector
    q_0_quat = [qt_base; q_0(17:end)];
end

== matlab function POSITION CONTROLLER (IK)/Integration Based InverseKinematics/InverseKinematics Integration/Rewirte the Base Pose as Transf Matrix ==
  data: q_ikin_quat input double; q_ikin output double
function q_ikin = fromQuaternionsToTransfMatr(q_ikin_quat)

    % define the base pose in quaternions
    q_base           = q_ikin_quat(1:7);

    % define the transformation matrix
    w_H_b            = wbc.fromPosQuatToTransfMatr(q_base);

    % column-major serialization
    w_H_b_vectorized = w_H_b(:);

    % new state vector
    q_ikin           = [w_H_b_vectorized; q_ikin_quat(8:end)];
end
